simulink model "MaskKoshiLong"  (Simulink 7.9)
settings: Solver=ode45  StartTime=0.0  StopTime=100.0  RelTol=1e-3
libraries: simulink x2
settings Model: Creator=Mihail  LastModifiedBy=Mihail

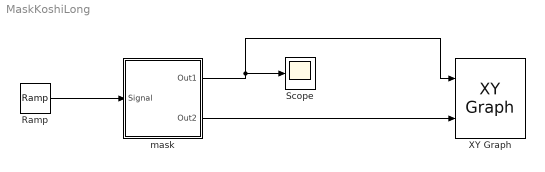
== system MaskKoshiLong ==
  Ramp : simulink/Sources/Ramp  slope=1  start=0  X0=1
  Scope : Scope
      settings: TimeRange=5  YMin=0  YMax=1000000
  XY Graph : simulink/Sinks/XY Graph  xmin=-50  xmax=50  ymin=-50  ymax=50  st=0.1
  mask : Subsystem  mask{a11=0, a12=1, a21=-4, a22=-4, f1=0, f2=u*cos(u), D1=-1, D2=1}
      mask prompts: a11 "A[1,1]"; a12 "A[1,2]"; a21 "A[2,1]"; a22 "A[2,2]"; f1 "F[1]"; f2 "F[2]"; D1 "Y(0)[1]"; D2 "Y(0)[2]"
  wires:
  Ramp/1 -> mask/1(Signal)
  mask/1(Out1) -> Scope/1, XY Graph/1
  mask/2(Out2) -> XY Graph/2

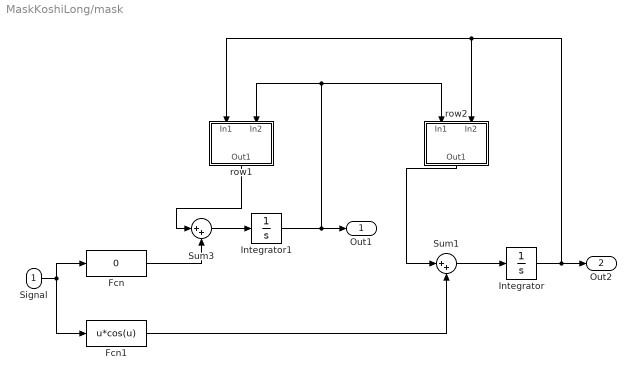
== system MaskKoshiLong/mask ==
  Signal : Inport
  " row1" : Subsystem
  Fcn : Fcn  Expr=0
  Fcn1 : Fcn  Expr=u*cos(u)
  Integrator : Integrator  InitialCondition=D2
  Integrator1 : Integrator  InitialCondition=D1
  Sum1 : Sum  Inputs=|++
  Sum3 : Sum  Inputs=|++
  "row2 " : Subsystem
  Out1 : Outport
  Out2 : Outport  Port=2
  wires:
  Signal/1 -> Fcn/1, Fcn1/1
  Fcn/1 -> Sum3/2
  Sum3/1 -> Integrator1/1
  Integrator1/1 -> Out1/1, " row1"/2(In2), "row2 "/1(In1)
  Fcn1/1 -> Sum1/2
  Sum1/1 -> Integrator/1
  Integrator/1 -> Out2/1, " row1"/1(In1), "row2 "/2(In2)
  "row2 "/1(Out1) -> Sum1/1
  " row1"/1(Out1) -> Sum3/1

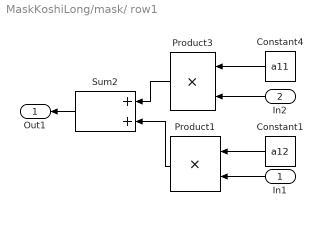
== system MaskKoshiLong/mask/ row1 ==
  In1 : Inport
  In2 : Inport  Port=2
  Constant1 : Constant  Value=a12
  Constant4 : Constant  Value=a11
  Product1 : Product
  Product3 : Product
  Sum2 : Sum  Inputs=|++
  Out1 : Outport
  wires:
  Product1/1 -> Sum2/2
  Product3/1 -> Sum2/1
  Constant1/1 -> Product1/1
  Constant4/1 -> Product3/1
  Sum2/1 -> Out1/1
  In1/1 -> Product1/2
  In2/1 -> Product3/2

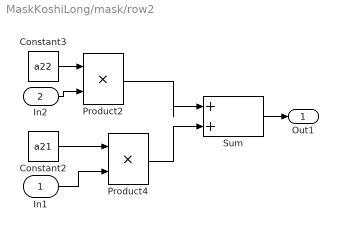
== system MaskKoshiLong/mask/row2  ==
  In1 : Inport
  In2 : Inport  Port=2
  Constant2 : Constant  Value=a21
  Constant3 : Constant  Value=a22
  Product2 : Product
  Product4 : Product
  Sum : Sum  Inputs=|++
  Out1 : Outport
  wires:
  Constant3/1 -> Product2/1
  Constant2/1 -> Product4/1
  Product2/1 -> Sum/1
  Product4/1 -> Sum/2
  Sum/1 -> Out1/1
  In1/1 -> Product4/2
  In2/1 -> Product2/2
